simulink model "OCKModel"  (R2017b)
settings: Solver=FixedStepAuto  StartTime=0.0  StopTime=sim.T  FixedStep=sim.Ts  RelTol=1e-3
PreLoadFcn:
  | preLoadCallback
StartFcn:
  | startCallback
StopFcn:
  | stopCallback
values from neighbouring files (symbols this model uses):
  p = simulationParametersClass    [preLoadCallback.m]
undefined symbols (not defined in the file or in its folder): env, faults, plant
libraries: lowLevel x24, controllers x1, simulink x1, controllerComponents x1, flowVariants x1
settings Model: SimulationMode=rapid-accelerator  PauseTimes=78.131  SnapshotBufferSize=2  SnapshotInterval=1  ExtModeTrigDuration=100  Creator=M.Cobb  LastModifiedBy=mitch
settings DataIOCC: SaveOutput=off  StateSaveName=tmp_raccel_xout
settings OptimizationCC: DefaultParameterBehavior=Inlined  EfficientMapNaN2IntZero=off
settings DebuggingCC: InheritedTsInSrcMsg=none  AllowedUnitSystems=SI,SI (extended)
settings HardwareCC: TargetBitPerPointer=64  TargetBitPerSizeT=64  TargetBitPerPtrDiffT=64  TargetLongLongMode=on  TargetIntDivRoundTo=Zero  TargetEndianess=LittleEndian  TargetWordSize=64  TargetHWDeviceType=MATLAB Host  ProdEqTarget=off
settings RTWCC: SystemTargetFile=raccel.tlc  TemplateMakefile=raccel_default_tmf  RTWVerbose=off  RTWUseSimCustomCode=on
settings CodeAppCC: GenerateComments=off  MaxIdLength=128  MangleLength=10  SimulinkBlockComments=off
settings RaccelTargetCC: GeneratePreprocessorConditionals=Use local settings  MultiInstanceERTCode=off  ENABLE_SLEXEC_SSBRIDGE=11  RTWCAPIParams=on

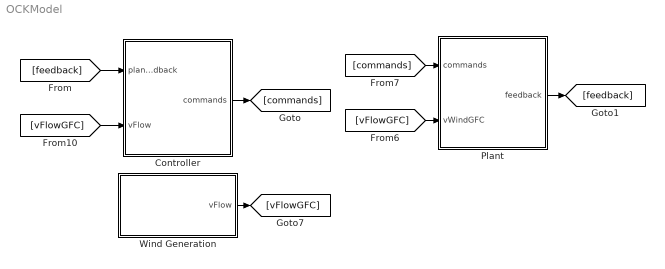
== system OCKModel ==
  Controller : Subsystem  Variant=on
  Plant : Subsystem
  Wind Generation : Subsystem
  wires:
  Wind Generation/1(vFlow) -> [vFlowGFC]
  [vFlowGFC] -> Plant/2(vWindGFC)
  [vFlowGFC] -> Controller/2(vFlow)
  Controller/1(commands) -> [commands]
  [commands] -> Plant/1(commands)
  Plant/1(feedback) -> [feedback]
  [feedback] -> Controller/1(plantFeedback)

== system OCKModel/Controller ==
  plantFeedback : Inport  OutDataTypeStr=Bus: busPlantFeedback
  vFlow : Inport  Port=2
  OCK Controller : controllers/OCK Controller  VariantControl=variantOCK
  commands : Outport  OutDataTypeStr=Bus: busControllerOutput

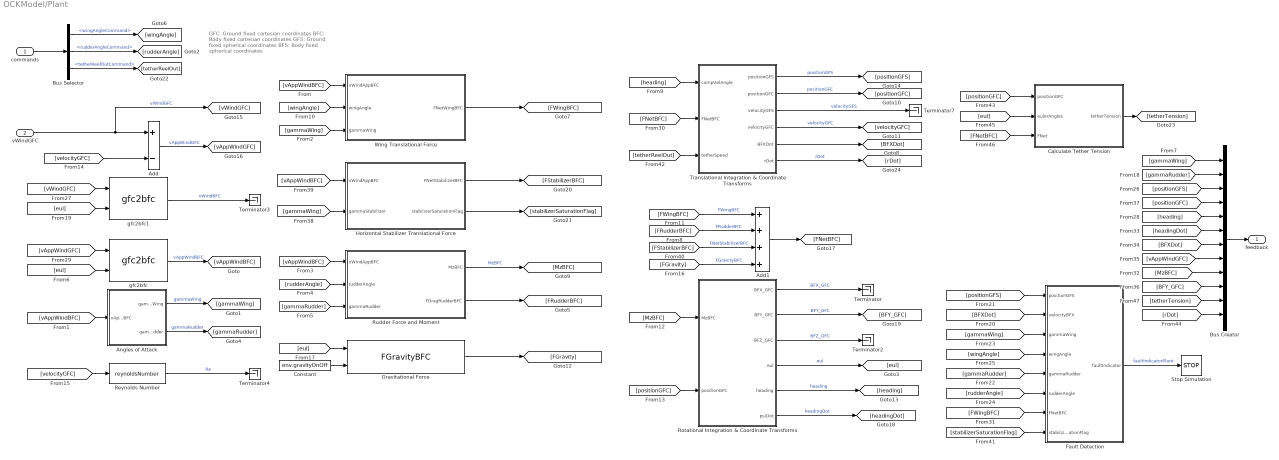
== system OCKModel/Plant ==
  note: GFC: Ground fixed cartesian coordinates
      | BFC:  Body fixed cartesian coordinates
      | GFS: Ground fixed spherical coordinates
      | BFS: Body fixed spherical coordinates
  commands : Inport  OutDataTypeStr=Bus: busControllerOutput
  vWindGFC : Inport  Port=2
  Add : Sum  Inputs=+-
  Add1 : Sum  Inputs=++++
  Angles of Attack : Subsystem
  Bus Selector : BusSelector  OutputSignals=wingAngleCommand,rudderAngleCommand,tetherReelOutCommand
  Bus Creator : BusCreator  Inputs=12  OutDataTypeStr=Bus: busPlantFeedback
  Calculate Tether Tension : Subsystem
  Constant : Constant  Value=env.gravityOnOff
  Fault Detection : Subsystem
  Gravitational Force : lowLevel/FGravityBFC
  Horizontal Stabilizer Translational Force : Subsystem
  Reynolds Number : lowLevel/reynoldsNumber
  Rotational Integration & Coordinate Transforms : Subsystem
  Rudder Force and Moment : Subsystem
  Stop Simulation : Stop
  Terminator{,2..4,7} (5 alike) : Terminator
  Translational Integration & Coordinate Transforms : Subsystem
  Wing Translational Force : Subsystem
  gfc2bfc : lowLevel/gfc2bfc
  gfc2bfc1 : lowLevel/gfc2bfc
  feedback : Outport  OutDataTypeStr=Bus: busPlantFeedback
  wires:
  vWindGFC/1 -> [vWindGFC], Add/1  "vWindGFC"
  [vAppWindBFC] -> Angles of Attack/1(vAppWindBFC)
  Angles of Attack/1(gammaWing) -> [gammaWing]  "gammaWing"
  [vAppWindBFC] -> Wing Translational Force/1(vWindAppBFC)
  Add/1 -> [vAppWindGFC]  "vAppWindGFC"
  [vAppWindBFC] -> Rudder Force and Moment/1(vWindAppBFC)
  [rudderAngle] -> Rudder Force and Moment/2(rudderAngle)
  Translational Integration & Coordinate Transforms/2(positionGFC) -> [positionGFC]  "positionGFC"
  Rudder Force and Moment/2(FDragRudderBFC) -> [FRudderBFC]
  [gammaWing] -> Wing Translational Force/3(gammaWing)
  [heading] -> Translational Integration & Coordinate Transforms/1(compVelAngle)
  Angles of Attack/2(gammaRudder) -> [gammaRudder]  "gammaRudder"
  [gammaRudder] -> Rudder Force and Moment/3(gammaRudder)
  Wing Translational Force/1(FNetWingBFC) -> [FWingBFC]
  [wingAngle] -> Wing Translational Force/2(wingAngle)
  [FNetBFC] -> Translational Integration & Coordinate Transforms/2(FNetBFC)
  Rudder Force and Moment/1(MzBFC) -> [MzBFC]  "MzBFC"
  [MzBFC] -> Rotational Integration & Coordinate Transforms/1(MzBFC)
  [positionGFC] -> Rotational Integration & Coordinate Transforms/2(positionGFC)
  Rotational Integration & Coordinate Transforms/4(eul) -> [eul]  "eul"
  Rotational Integration & Coordinate Transforms/1(BFX_GFC) -> Terminator/1  "BFX_GFC"
  Rotational Integration & Coordinate Transforms/2(BFY_GFC) -> [BFY_GFC]  "BFY_GFC"
  Rotational Integration & Coordinate Transforms/3(BFZ_GFC) -> Terminator2/1  "BFZ_GFC"
  Translational Integration & Coordinate Transforms/4(velocityGFC) -> [velocityGFC]  "velocityGFC"
  [velocityGFC] -> Add/2
  [velocityGFC] -> Reynolds Number/1
  Reynolds Number/1 -> Terminator4/1  "Re"
  Gravitational Force/1 -> [FGravity]
  [eul] -> Gravitational Force/1
  Translational Integration & Coordinate Transforms/1(positionGFS) -> [positionGFS]  "positionGFS"
  Translational Integration & Coordinate Transforms/3(velocityGFS) -> Terminator7/1  "velocityGFS"
  [eul] -> gfc2bfc1/2
  gfc2bfc1/1 -> Terminator3/1  "vWindBFC"
  Rotational Integration & Coordinate Transforms/5(heading) -> [heading]  "heading"
  Constant/1 -> Gravitational Force/2
  Translational Integration & Coordinate Transforms/5(BFXDot) -> [BFXDot]
  [BFXDot] -> Fault Detection/2(velocityBFX)
  [positionGFS] -> Fault Detection/1(positionGFS)
  Fault Detection/1(faultIndicator) -> Stop Simulation/1  "faultIndicatorPlant"
  [gammaRudder] -> Fault Detection/5(gammaRudder)
  [gammaWing] -> Fault Detection/3(gammaWing)
  [rudderAngle] -> Fault Detection/6(rudderAngle)
  [wingAngle] -> Fault Detection/4(wingAngle)
  [vWindGFC] -> gfc2bfc1/1
  gfc2bfc/1 -> [vAppWindBFC]  "vAppWindBFC"
  [eul] -> gfc2bfc/2
  [vAppWindGFC] -> gfc2bfc/1
  [FWingBFC] -> Add1/1  "FWingBFC"
  [FRudderBFC] -> Add1/2  "FRudderBFC"
  Add1/1 -> [FNetBFC]
  [FWingBFC] -> Fault Detection/7(FNetBFC)
  commands/1 -> Bus Selector/1
  Bus Selector/1 -> [wingAngle]  "<wingAngleCommand>"
  Bus Selector/2 -> [rudderAngle]  "<rudderAngleCommand>"
  [gammaWing] -> Bus Creator/1
  Bus Creator/1 -> feedback/1
  [gammaRudder] -> Bus Creator/2
  [positionGFS] -> Bus Creator/3
  Rotational Integration & Coordinate Transforms/6(psiDot) -> [headingDot]  "headingDot"
  [BFY_GFC] -> Bus Creator/10
  [MzBFC] -> Bus Creator/9
  [vAppWindGFC] -> Bus Creator/8
  [headingDot] -> Bus Creator/6
  [heading] -> Bus Creator/5
  [BFXDot] -> Bus Creator/7
  [positionGFC] -> Bus Creator/4
  [gammaWing] -> Horizontal Stabilizer Translational Force/2(gammaStabilizer)
  [vAppWindBFC] -> Horizontal Stabilizer Translational Force/1(vWindAppBFC)
  Horizontal Stabilizer Translational Force/1(FNetStabilizerBFC) -> [FStabilizerBFC]
  [FStabilizerBFC] -> Add1/3  "FNetStabilizerBFC"
  [FGravity] -> Add1/4  "FGravityBFC"
  Horizontal Stabilizer Translational Force/2(stabilizerSaturationFlag) -> [stabilizerSaturationFlag]
  [stabilizerSaturationFlag] -> Fault Detection/8(stabilizerSaturationFlag)
  Bus Selector/3 -> [tetherReelOut]  "<tetherReelOutCommand>"
  [tetherReelOut] -> Translational Integration & Coordinate Transforms/3(tetherSpeed)
  [positionGFC] -> Calculate Tether Tension/1(positionGFC)
  [eul] -> Calculate Tether Tension/2(eulerAngles)
  [FNetBFC] -> Calculate Tether Tension/3(FNet)
  [tetherTension] -> Bus Creator/11
  Calculate Tether Tension/1(tetherTension) -> [tetherTension]
  Translational Integration & Coordinate Transforms/6(rDot) -> [rDot]  "rDot"
  [rDot] -> Bus Creator/12

== system OCKModel/Wind Generation ==
  Variant Subsystem : Subsystem  Variant=on
  vFlow : Outport
  wires:
  Variant Subsystem/1(vFlowGFC) -> vFlow/1  "vFlowGFC"

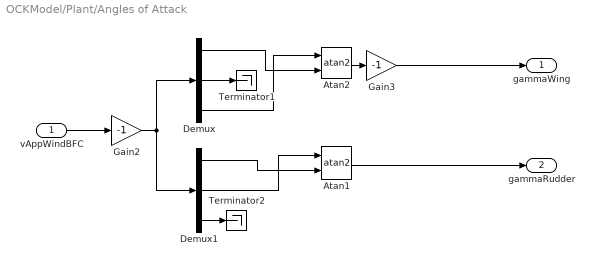
== system OCKModel/Plant/Angles of Attack ==
  vAppWindBFC : Inport
  Atan1 : Trigonometry  Operator=atan2
  Atan2 : Trigonometry  Operator=atan2
  Demux : Demux  Outputs=3
  Demux1 : Demux  Outputs=3
  Gain2 : Gain  Gain=-1
  Gain3 : Gain  Gain=-1
  Terminator1 : Terminator
  Terminator2 : Terminator
  gammaWing : Outport
  gammaRudder : Outport  Port=2
  wires:
  vAppWindBFC/1 -> Gain2/1
  Demux/1 -> Atan2/2
  Atan2/1 -> Gain3/1
  Demux/3 -> Atan2/1
  Demux/2 -> Terminator1/1
  Demux1/3 -> Terminator2/1
  Gain2/1 -> Demux1/1, Demux/1
  Atan1/1 -> gammaRudder/1
  Gain3/1 -> gammaWing/1
  Demux1/1 -> Atan1/2
  Demux1/2 -> Atan1/1

== system OCKModel/Plant/Calculate Tether Tension ==
  positionGFC : Inport
  eulerAngles : Inport  Port=2
  FNet : Inport  Port=3
  Dot Product : DotProduct  InputSameDT=on  OutDataTypeStr=Inherit: Inherit via internal rule
  gfc2bfc : lowLevel/gfc2bfc
  normalize : lowLevel/normalize
  tetherTension : Outport
  wires:
  positionGFC/1 -> normalize/1
  normalize/1 -> gfc2bfc/1
  eulerAngles/1 -> gfc2bfc/2
  FNet/1 -> Dot Product/2
  gfc2bfc/1 -> Dot Product/1
  Dot Product/1 -> tetherTension/1  "tetherTension"

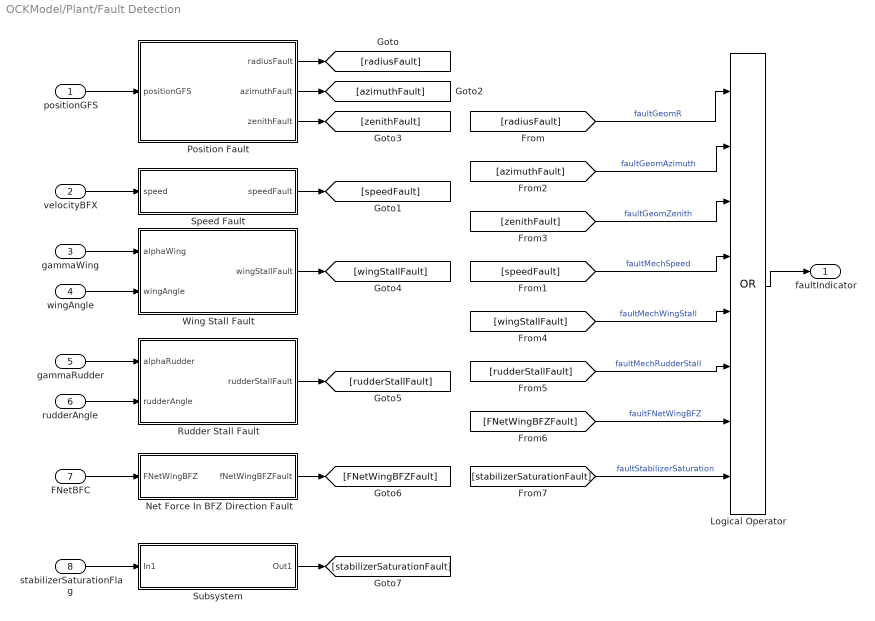
== system OCKModel/Plant/Fault Detection ==
  positionGFS : Inport
  velocityBFX : Inport  Port=2
  gammaWing : Inport  Port=3
  wingAngle : Inport  Port=4
  gammaRudder : Inport  Port=5
  rudderAngle : Inport  Port=6
  FNetBFC : Inport  Port=7
  stabilizerSaturationFlag : Inport  Port=8
  Logical Operator : Logic  Operator=OR  Inputs=8  AllPortsSameDT=off  OutDataTypeStr=boolean
  Net Force In BFZ Direction Fault : Subsystem
  Position Fault : Subsystem
  Rudder Stall Fault : Subsystem
  Speed Fault : Subsystem
  Subsystem : Subsystem
  Wing Stall Fault : Subsystem
  faultIndicator : Outport
  wires:
  positionGFS/1 -> Position Fault/1(positionGFS)
  Logical Operator/1 -> faultIndicator/1
  Speed Fault/1(speedFault) -> [speedFault]
  velocityBFX/1 -> Speed Fault/1(speed)
  [radiusFault] -> Logical Operator/1  "faultGeomR"
  [speedFault] -> Logical Operator/4  "faultMechSpeed"
  [azimuthFault] -> Logical Operator/2  "faultGeomAzimuth"
  [zenithFault] -> Logical Operator/3  "faultGeomZenith"
  Wing Stall Fault/1(wingStallFault) -> [wingStallFault]
  gammaWing/1 -> Wing Stall Fault/1(alphaWing)
  gammaRudder/1 -> Rudder Stall Fault/1(alphaRudder)
  [wingStallFault] -> Logical Operator/5  "faultMechWingStall"
  [rudderStallFault] -> Logical Operator/6  "faultMechRudderStall"
  wingAngle/1 -> Wing Stall Fault/2(wingAngle)
  rudderAngle/1 -> Rudder Stall Fault/2(rudderAngle)
  Rudder Stall Fault/1(rudderStallFault) -> [rudderStallFault]
  Position Fault/1(radiusFault) -> [radiusFault]
  Position Fault/2(azimuthFault) -> [azimuthFault]
  Position Fault/3(zenithFault) -> [zenithFault]
  Net Force In BFZ Direction Fault/1(fNetWingBFZFault) -> [FNetWingBFZFault]
  FNetBFC/1 -> Net Force In BFZ Direction Fault/1(FNetWingBFZ)
  [FNetWingBFZFault] -> Logical Operator/7  "faultFNetWingBFZ"
  [stabilizerSaturationFault] -> Logical Operator/8  "faultStabilizerSaturation"
  stabilizerSaturationFlag/1 -> Subsystem/1(In1)
  Subsystem/1(Out1) -> [stabilizerSaturationFault]

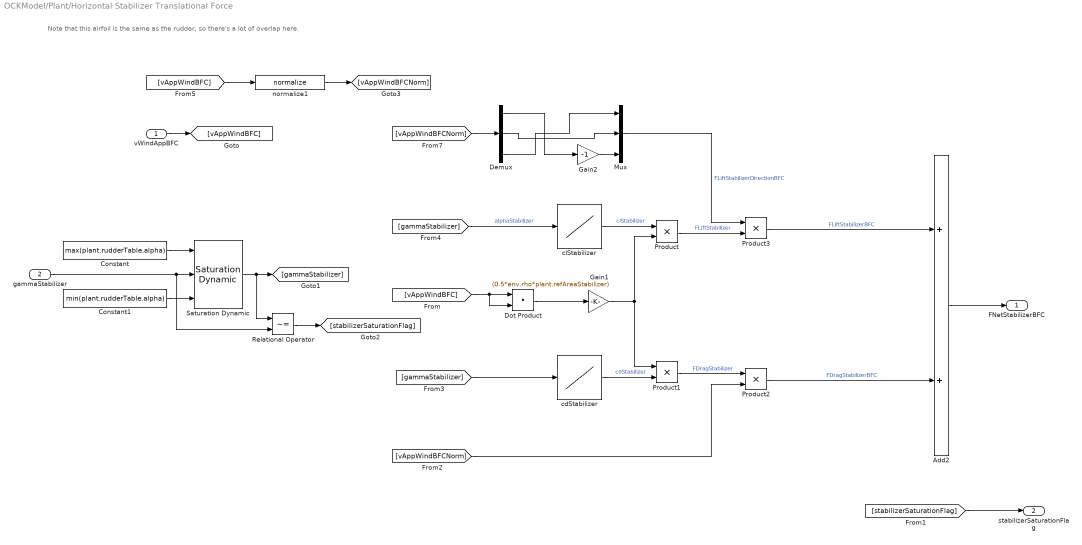
== system OCKModel/Plant/Horizontal Stabilizer Translational Force ==
  note: Note that this airfoil is the same as the rudder, so there's a lot of overlap here.
  vWindAppBFC : Inport
  gammaStabilizer : Inport  Port=2
  Add2 : Sum
  Constant : Constant  Value=max(plant.rudderTable.alpha)
  Constant1 : Constant  Value=min(plant.rudderTable.alpha)
  Demux : Demux  Outputs=3
  Dot Product : DotProduct  InputSameDT=on  OutDataTypeStr=Inherit: Inherit via internal rule
  Gain1 : Gain  Gain=(0.5*env.rho*plant.refAreaStabilizer)
  Gain2 : Gain  Gain=-1
  Mux : Mux  Inputs=3
  Product{,1..3} (4 alike) : Product
  Relational Operator : RelationalOperator  Operator=~=  OutDataTypeStr=boolean  RndMeth=Simplest
  Saturation Dynamic : simulink/Discontinuities/Saturation Dynamic  OutMin=[]  OutMax=[]  OutDataTypeStr=Inherit: Same as second input  OutDataType=fixdt(1, 16)  OutScaling=2^-10  DoSatur=off
  cdStabilizer : Lookup_n-D  NumberOfTableDimensions=1  BreakpointsForDimension1=plant.rudderTable.alpha  Table=plant.rudderTable.cd  InternalRulePriority=Speed  RndMeth=Simplest  InputSameDT=on
  clStabilizer : Lookup_n-D  NumberOfTableDimensions=1  BreakpointsForDimension1=plant.rudderTable.alpha  Table=plant.rudderTable.cl  InternalRulePriority=Speed  RndMeth=Simplest  InputSameDT=on
  normalize1 : lowLevel/normalize
  FNetStabilizerBFC : Outport
  stabilizerSaturationFlag : Outport  Port=2
  wires:
  Product1/1 -> Product2/1  "FDragStabilizer"
  Product2/1 -> Add2/2  "FDragStabilizerBFC"
  Product/1 -> Product3/2  "FLiftStabilizer"
  Product3/1 -> Add2/1  "FLiftStabilizerBFC"
  Dot Product/1 -> Gain1/1
  clStabilizer/1 -> Product/1  "clStabilizer"
  [vAppWindBFC] -> Dot Product/1, Dot Product/2
  Gain1/1 -> Product/2, Product1/1
  cdStabilizer/1 -> Product1/2  "cdStabilizer"
  vWindAppBFC/1 -> [vAppWindBFC]
  gammaStabilizer/1 -> Relational Operator/2, Saturation Dynamic/2
  Demux/2 -> Mux/2
  Demux/1 -> Gain2/1
  Mux/1 -> Product3/1  "FLiftStabilizerDirectionBFC"
  Demux/3 -> Mux/1
  [vAppWindBFC] -> normalize1/1
  normalize1/1 -> [vAppWindBFCNorm]
  [vAppWindBFCNorm] -> Demux/1
  [vAppWindBFCNorm] -> Product2/2
  Gain2/1 -> Mux/3
  [gammaStabilizer] -> cdStabilizer/1
  [gammaStabilizer] -> clStabilizer/1  "alphaStabilizer"
  Saturation Dynamic/1 -> Relational Operator/1, [gammaStabilizer]
  Constant/1 -> Saturation Dynamic/1
  Constant1/1 -> Saturation Dynamic/3
  Relational Operator/1 -> [stabilizerSaturationFlag]
  [stabilizerSaturationFlag] -> stabilizerSaturationFlag/1
  Add2/1 -> FNetStabilizerBFC/1

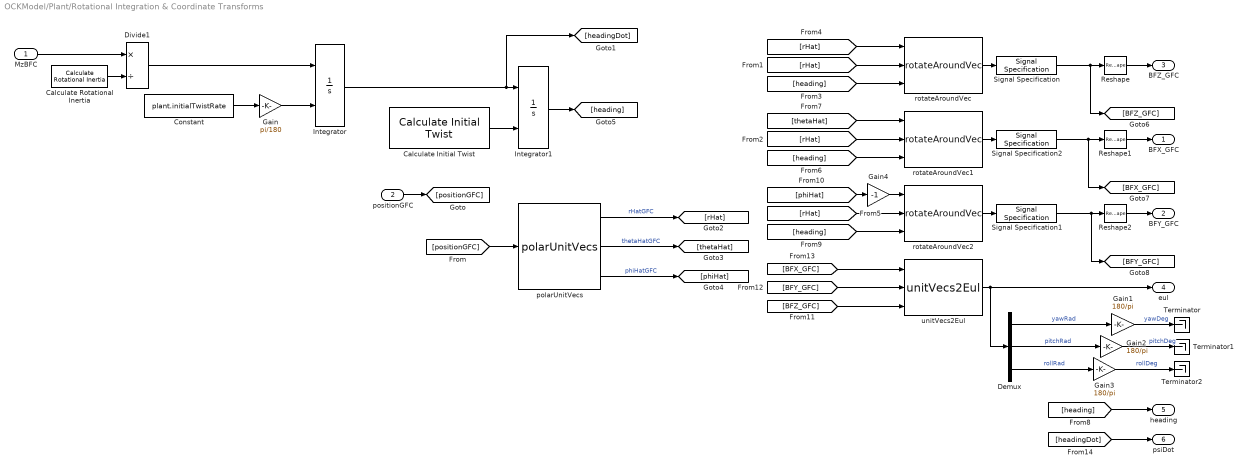
== system OCKModel/Plant/Rotational Integration & Coordinate Transforms ==
  MzBFC : Inport  PortDimensions=1
  positionGFC : Inport  Port=2
  Calculate Rotational Inertia : lowLevel/Calculate Rotational Inertia
  Calculate Initial Twist : controllerComponents/Calculate Initial Twist
  Constant : Constant  Value=plant.initialTwistRate
  Demux : Demux  Outputs=3
  Divide1 : Product  Inputs=*/
  Gain : Gain  Gain=pi/180
  Gain1 : Gain  Gain=180/pi
  Gain2 : Gain  Gain=180/pi
  Gain3 : Gain  Gain=180/pi
  Gain4 : Gain  Gain=-1
  Integrator : Integrator  InitialConditionSource=external  InitialCondition=plant.initialTwistRate
  Integrator1 : Integrator  InitialConditionSource=external  InitialCondition=plant.initialTwist
  Reshape : Reshape  OutputDimensions=[3 1]
  Reshape1 : Reshape  OutputDimensions=[3 1]
  Reshape2 : Reshape  OutputDimensions=[3 1]
  Signal Specification : SignalSpecification  Dimensions=[1 3]
  Signal Specification1 : SignalSpecification  Dimensions=[1 3]
  Signal Specification2 : SignalSpecification  Dimensions=[1 3]
  Terminator : Terminator
  Terminator1 : Terminator
  Terminator2 : Terminator
  polarUnitVecs : lowLevel/polarUnitVecs
  rotateAroundVec : lowLevel/rotateAroundVec
  rotateAroundVec1 : lowLevel/rotateAroundVec
  rotateAroundVec2 : lowLevel/rotateAroundVec
  unitVecs2Eul : lowLevel/unitVecs2Eul
  BFX_GFC : Outport
  BFY_GFC : Outport  Port=2
  BFZ_GFC : Outport  Port=3
  eul : Outport  Port=4  PortDimensions=3
  heading : Outport  Port=5  PortDimensions=1
  psiDot : Outport  Port=6  PortDimensions=1
  wires:
  MzBFC/1 -> Divide1/1
  Integrator/1 -> [headingDot], Integrator1/1
  positionGFC/1 -> [positionGFC]
  [positionGFC] -> polarUnitVecs/1
  polarUnitVecs/1 -> [rHat]  "rHatGFC"
  polarUnitVecs/2 -> [thetaHat]  "thetaHatGFC"
  polarUnitVecs/3 -> [phiHat]  "phiHatGFC"
  Integrator1/1 -> [heading]
  [heading] -> rotateAroundVec/3
  [rHat] -> rotateAroundVec/1
  [rHat] -> rotateAroundVec/2
  [thetaHat] -> rotateAroundVec1/1
  [heading] -> rotateAroundVec1/3
  [rHat] -> rotateAroundVec1/2
  [phiHat] -> Gain4/1
  [heading] -> rotateAroundVec2/3
  [rHat] -> rotateAroundVec2/2
  unitVecs2Eul/1 -> Demux/1, eul/1
  [BFZ_GFC] -> unitVecs2Eul/3
  [BFY_GFC] -> unitVecs2Eul/2
  [BFX_GFC] -> unitVecs2Eul/1
  Demux/3 -> Gain3/1  "rollRad"
  Demux/2 -> Gain2/1  "pitchRad"
  Demux/1 -> Gain1/1  "yawRad"
  Gain1/1 -> Terminator/1  "yawDeg"
  Gain2/1 -> Terminator1/1  "pitchDeg"
  Gain3/1 -> Terminator2/1  "rollDeg"
  Gain4/1 -> rotateAroundVec2/1
  rotateAroundVec/1 -> Signal Specification/1
  rotateAroundVec1/1 -> Signal Specification2/1
  rotateAroundVec2/1 -> Signal Specification1/1
  Signal Specification/1 -> Reshape/1, [BFZ_GFC]
  Signal Specification2/1 -> [BFX_GFC], Reshape1/1
  Signal Specification1/1 -> [BFY_GFC], Reshape2/1
  Reshape/1 -> BFZ_GFC/1
  Reshape1/1 -> BFX_GFC/1
  Reshape2/1 -> BFY_GFC/1
  [heading] -> heading/1
  [headingDot] -> psiDot/1
  Calculate Initial Twist/1 -> Integrator1/2
  Calculate Rotational Inertia/1 -> Divide1/2
  Divide1/1 -> Integrator/1
  Constant/1 -> Gain/1
  Gain/1 -> Integrator/2

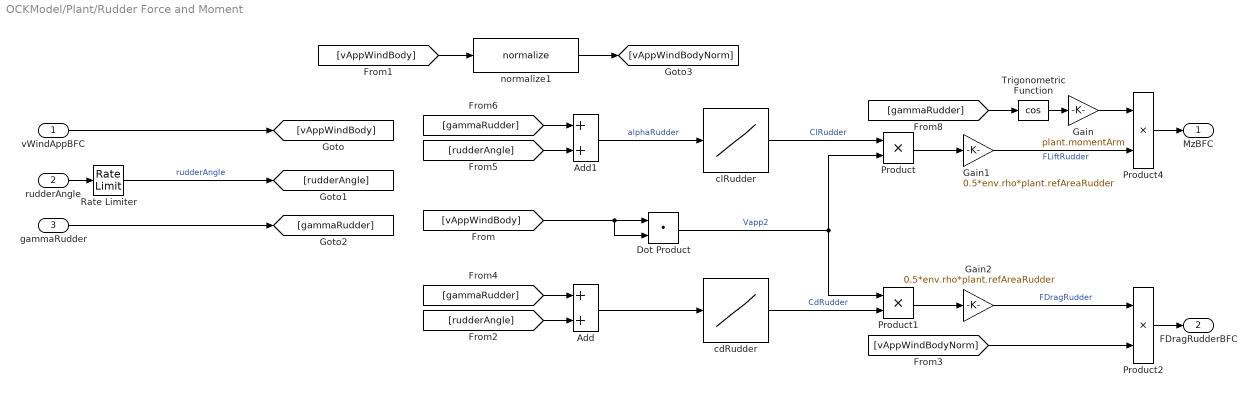
== system OCKModel/Plant/Rudder Force and Moment ==
  vWindAppBFC : Inport
  rudderAngle : Inport  Port=2
  gammaRudder : Inport  Port=3
  Add : Sum
  Add1 : Sum
  Dot Product : DotProduct  InputSameDT=on  OutDataTypeStr=Inherit: Inherit via internal rule
  Gain : Gain  Gain=plant.momentArm
  Gain1 : Gain  Gain=0.5*env.rho*plant.refAreaRudder
  Gain2 : Gain  Gain=0.5*env.rho*plant.refAreaRudder
  Product{,1..2,4} (4 alike) : Product
  Rate Limiter : RateLimiter  RisingSlewLimit=plant.rudderAngleRateLimit*pi/180  FallingSlewLimit=-plant.rudderAngleRateLimit*pi/180  SampleTimeMode=inherited
  Trigonometric Function : Trigonometry  Operator=cos
  cdRudder : Lookup_n-D  NumberOfTableDimensions=1  BreakpointsForDimension1=plant.rudderTable.alpha  Table=plant.rudderTable.cd  InternalRulePriority=Speed  RndMeth=Simplest  InputSameDT=on
  clRudder : Lookup_n-D  NumberOfTableDimensions=1  BreakpointsForDimension1=plant.rudderTable.alpha  Table=plant.rudderTable.cl  InternalRulePriority=Speed  RndMeth=Simplest  InputSameDT=on
  normalize1 : lowLevel/normalize
  MzBFC : Outport
  FDragRudderBFC : Outport  Port=2
  wires:
  clRudder/1 -> Product/1  "ClRudder"
  [vAppWindBody] -> Dot Product/2, Dot Product/1
  Dot Product/1 -> Product1/1, Product/2  "Vapp2"
  vWindAppBFC/1 -> [vAppWindBody]
  rudderAngle/1 -> Rate Limiter/1
  Product/1 -> Gain1/1
  cdRudder/1 -> Product1/2  "CdRudder"
  Product1/1 -> Gain2/1
  Gain2/1 -> Product2/1  "FDragRudder"
  [vAppWindBodyNorm] -> Product2/2
  gammaRudder/1 -> [gammaRudder]
  [rudderAngle] -> Add/2
  [gammaRudder] -> Add/1
  Add/1 -> cdRudder/1
  [rudderAngle] -> Add1/2
  [gammaRudder] -> Add1/1
  Add1/1 -> clRudder/1  "alphaRudder"
  Gain1/1 -> Product4/2  "FLiftRudder"
  [vAppWindBody] -> normalize1/1
  normalize1/1 -> [vAppWindBodyNorm]
  Product2/1 -> FDragRudderBFC/1
  [gammaRudder] -> Trigonometric Function/1
  Product4/1 -> MzBFC/1
  Trigonometric Function/1 -> Gain/1
  Gain/1 -> Product4/1
  Rate Limiter/1 -> [rudderAngle]  "rudderAngle"

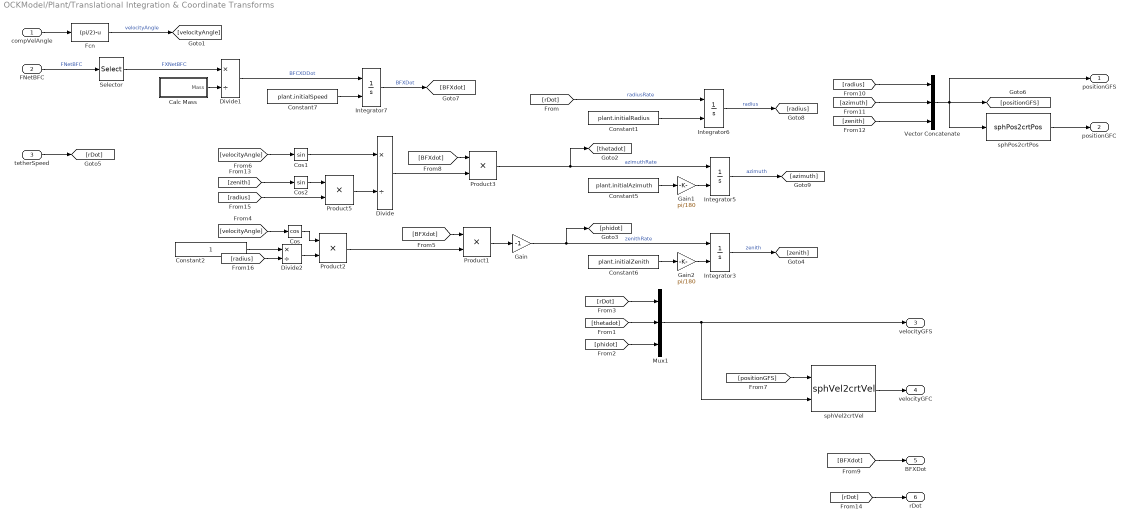
== system OCKModel/Plant/Translational Integration & Coordinate Transforms ==
  compVelAngle : Inport
  FNetBFC : Inport  Port=2
  tetherSpeed : Inport  Port=3
  Calc Mass : Subsystem
  Constant1 : Constant  Value=plant.initialRadius
  Constant2 : Constant
  Constant5 : Constant  Value=plant.initialAzimuth
  Constant6 : Constant  Value=plant.initialZenith
  Constant7 : Constant  Value=plant.initialSpeed
  Cos : Trigonometry  Operator=cos
  Cos1 : Trigonometry
  Cos2 : Trigonometry
  Divide : Product  Inputs=*/
  Divide1 : Product  Inputs=*/
  Divide2 : Product  Inputs=*/
  Fcn : Fcn  Expr=(pi/2)-u
  Gain : Gain  Gain=-1
  Gain1 : Gain  Gain=pi/180
  Gain2 : Gain  Gain=pi/180
  Integrator3 : Integrator  InitialConditionSource=external  InitialCondition=p.initPositionGFS(3)
  Integrator5 : Integrator  InitialConditionSource=external  InitialCondition=p.initPositionGFS(2)
  Integrator6 : Integrator  InitialConditionSource=external  InitialCondition=p.initPositionGFS(1)
  Integrator7 : Integrator  InitialConditionSource=external  InitialCondition=p.initVelocity
  Mux1 : Mux  Inputs=3
  Product{1..3,5} (4 alike) : Product
  Selector : Selector  InputPortWidth=3  IndexOptions=Index vector (dialog)  Indices=1  OutputSizes=1
  Vector Concatenate : Concatenate  NumInputs=3
  sphPos2crtPos : lowLevel/sphPos2crtPos
  sphVel2crtVel : lowLevel/sphVel2crtVel
  positionGFS : Outport  PortDimensions=3
  positionGFC : Outport  Port=2  PortDimensions=3
  velocityGFS : Outport  Port=3  PortDimensions=3
  velocityGFC : Outport  Port=4  PortDimensions=3
  BFXDot : Outport  Port=5
  rDot : Outport  Port=6
  wires:
  Gain/1 -> [phidot], Integrator3/1  "zenithRate"
  Integrator5/1 -> [azimuth]  "azimuth"
  Product3/1 -> [thetadot], Integrator5/1  "azimuthRate"
  Integrator3/1 -> [zenith]  "zenith"
  sphPos2crtPos/1 -> positionGFC/1
  sphVel2crtVel/1 -> velocityGFC/1
  [rDot] -> Mux1/1
  [thetadot] -> Mux1/2
  [phidot] -> Mux1/3
  FNetBFC/1 -> Selector/1  "FNetBFC"
  compVelAngle/1 -> Fcn/1
  Integrator6/1 -> [radius]  "radius"
  Mux1/1 -> sphVel2crtVel/2, velocityGFS/1
  [rDot] -> Integrator6/1  "radiusRate"
  [positionGFS] -> sphVel2crtVel/1
  Fcn/1 -> [velocityAngle]  "velocityAngle"
  [BFXdot] -> Product3/1
  [velocityAngle] -> Cos1/1
  Divide/1 -> Product3/2
  Cos1/1 -> Divide/1
  [radius] -> Product5/2
  [zenith] -> Cos2/1
  Cos2/1 -> Product5/1
  Product5/1 -> Divide/2
  [BFXdot] -> Product1/1
  [velocityAngle] -> Cos/1
  Product2/1 -> Product1/2
  Cos/1 -> Product2/1
  Divide2/1 -> Product2/2
  Product1/1 -> Gain/1
  Integrator7/1 -> [BFXdot]  "BFXDot"
  Divide1/1 -> Integrator7/1  "BFCXDDot"
  [BFXdot] -> BFXDot/1
  Constant1/1 -> Integrator6/2
  Constant5/1 -> Gain1/1
  Vector Concatenate/1 -> [positionGFS], positionGFS/1, sphPos2crtPos/1
  [radius] -> Vector Concatenate/1
  [azimuth] -> Vector Concatenate/2
  [zenith] -> Vector Concatenate/3
  Constant6/1 -> Gain2/1
  Gain1/1 -> Integrator5/2
  Gain2/1 -> Integrator3/2
  Constant7/1 -> Integrator7/2
  tetherSpeed/1 -> [rDot]
  Selector/1 -> Divide1/1  "FXNetBFC"
  Calc Mass/1(Mass) -> Divide1/2
  [rDot] -> rDot/1
  [radius] -> Divide2/2
  Constant2/1 -> Divide2/1

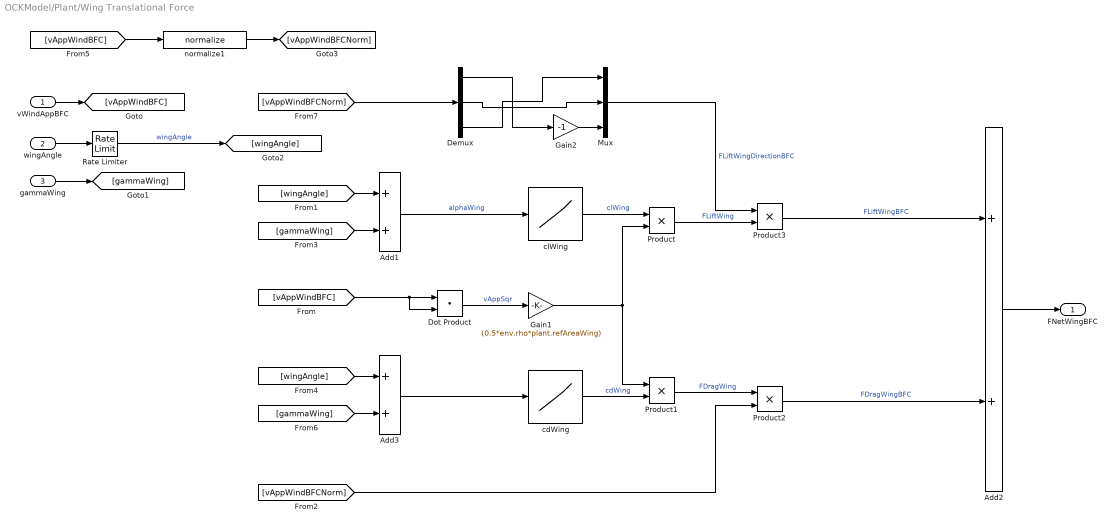
== system OCKModel/Plant/Wing Translational Force ==
  vWindAppBFC : Inport
  wingAngle : Inport  Port=2
  gammaWing : Inport  Port=3
  Add1 : Sum
  Add2 : Sum
  Add3 : Sum
  Demux : Demux  Outputs=3
  Dot Product : DotProduct  InputSameDT=on  OutDataTypeStr=Inherit: Inherit via internal rule
  Gain1 : Gain  Gain=(0.5*env.rho*plant.refAreaWing)
  Gain2 : Gain  Gain=-1
  Mux : Mux  Inputs=3
  Product{,1..3} (4 alike) : Product
  Rate Limiter : RateLimiter  RisingSlewLimit=plant.wingAngleRateLimit*pi/180  FallingSlewLimit=-plant.wingAngleRateLimit*pi/180  SampleTimeMode=inherited
  cdWing : Lookup_n-D  NumberOfTableDimensions=1  BreakpointsForDimension1=plant.wingTable.alpha  Table=plant.wingTable.cd  InternalRulePriority=Speed  RndMeth=Simplest  InputSameDT=on
  clWing : Lookup_n-D  NumberOfTableDimensions=1  BreakpointsForDimension1=plant.wingTable.alpha  Table=plant.wingTable.cl  InternalRulePriority=Speed  RndMeth=Simplest  InputSameDT=on
  normalize1 : lowLevel/normalize
  FNetWingBFC : Outport
  wires:
  Product1/1 -> Product2/1  "FDragWing"
  Product2/1 -> Add2/2  "FDragWingBFC"
  Product/1 -> Product3/2  "FLiftWing"
  Product3/1 -> Add2/1  "FLiftWingBFC"
  Dot Product/1 -> Gain1/1  "vAppSqr"
  clWing/1 -> Product/1  "clWing"
  [vAppWindBFC] -> Dot Product/2, Dot Product/1
  Gain1/1 -> Product/2, Product1/1
  cdWing/1 -> Product1/2  "cdWing"
  vWindAppBFC/1 -> [vAppWindBFC]
  Add2/1 -> FNetWingBFC/1
  gammaWing/1 -> [gammaWing]
  wingAngle/1 -> Rate Limiter/1
  [wingAngle] -> Add3/1
  [gammaWing] -> Add3/2
  Demux/1 -> Gain2/1
  Mux/1 -> Product3/1  "FLiftWingDirectionBFC"
  Demux/3 -> Mux/1
  [vAppWindBFC] -> normalize1/1
  normalize1/1 -> [vAppWindBFCNorm]
  [vAppWindBFCNorm] -> Demux/1
  [vAppWindBFCNorm] -> Product2/2
  Gain2/1 -> Mux/3
  Add3/1 -> cdWing/1
  [wingAngle] -> Add1/1
  [gammaWing] -> Add1/2
  Add1/1 -> clWing/1  "alphaWing"
  Rate Limiter/1 -> [wingAngle]  "wingAngle"
  Demux/2 -> Mux/2

== system OCKModel/Wind Generation/Variant Subsystem ==
  Constant Wind : flowVariants/Constant Wind  VariantControl=variantConstant
  vFlowGFC : Outport

== system OCKModel/Plant/Fault Detection/Net Force In BFZ Direction Fault ==
  note: If net force in body fixed Z direction is zero or negative
  FNetWingBFZ : Inport
  Constant10 : Constant  Value=faults.forceZHigh
  Constant11 : Constant  Value=faults.forceZEnable
  Constant9 : Constant  Value=faults.forceZLow
  Out Of Bounds Fault : lowLevel/Out Of Bounds Fault
  Selector : Selector  InputPortWidth=3  IndexOptions=Index vector (dialog)  Indices=3  OutputSizes=1
  fNetWingBFZFault : Outport
  wires:
  FNetWingBFZ/1 -> Selector/1
  Selector/1 -> Out Of Bounds Fault/1
  Constant9/1 -> Out Of Bounds Fault/2
  Constant10/1 -> Out Of Bounds Fault/3
  Constant11/1 -> Out Of Bounds Fault/4
  Out Of Bounds Fault/1 -> fNetWingBFZFault/1

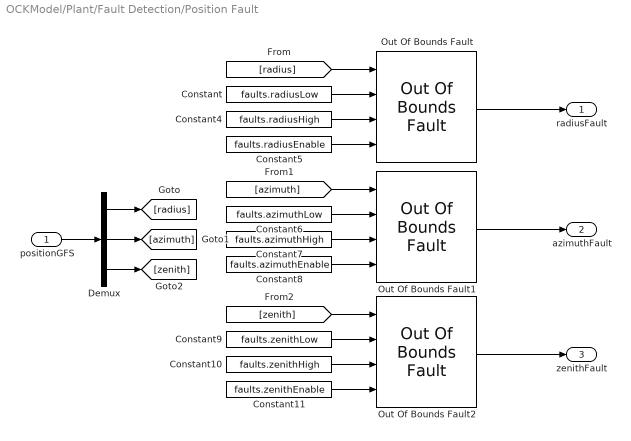
== system OCKModel/Plant/Fault Detection/Position Fault ==
  positionGFS : Inport
  Constant : Constant  Value=faults.radiusLow
  Constant10 : Constant  Value=faults.zenithHigh
  Constant11 : Constant  Value=faults.zenithEnable
  Constant4 : Constant  Value=faults.radiusHigh
  Constant5 : Constant  Value=faults.radiusEnable
  Constant6 : Constant  Value=faults.azimuthLow
  Constant7 : Constant  Value=faults.azimuthHigh
  Constant8 : Constant  Value=faults.azimuthEnable
  Constant9 : Constant  Value=faults.zenithLow
  Demux : Demux  Outputs=3
  Out Of Bounds Fault : lowLevel/Out Of Bounds Fault
  Out Of Bounds Fault1 : lowLevel/Out Of Bounds Fault
  Out Of Bounds Fault2 : lowLevel/Out Of Bounds Fault
  radiusFault : Outport
  azimuthFault : Outport  Port=2
  zenithFault : Outport  Port=3
  wires:
  positionGFS/1 -> Demux/1
  Out Of Bounds Fault/1 -> radiusFault/1
  Out Of Bounds Fault1/1 -> azimuthFault/1
  Out Of Bounds Fault2/1 -> zenithFault/1
  Demux/1 -> [radius]
  Demux/2 -> [azimuth]
  Demux/3 -> [zenith]
  [radius] -> Out Of Bounds Fault/1
  [azimuth] -> Out Of Bounds Fault1/1
  [zenith] -> Out Of Bounds Fault2/1
  Constant/1 -> Out Of Bounds Fault/2
  Constant5/1 -> Out Of Bounds Fault/4
  Constant4/1 -> Out Of Bounds Fault/3
  Constant7/1 -> Out Of Bounds Fault1/3
  Constant6/1 -> Out Of Bounds Fault1/2
  Constant8/1 -> Out Of Bounds Fault1/4
  Constant9/1 -> Out Of Bounds Fault2/2
  Constant10/1 -> Out Of Bounds Fault2/3
  Constant11/1 -> Out Of Bounds Fault2/4

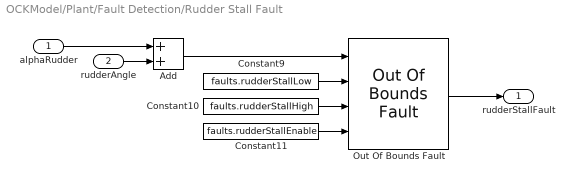
== system OCKModel/Plant/Fault Detection/Rudder Stall Fault ==
  alphaRudder : Inport
  rudderAngle : Inport  Port=2
  Add : Sum
  Constant10 : Constant  Value=faults.rudderStallHigh
  Constant11 : Constant  Value=faults.rudderStallEnable
  Constant9 : Constant  Value=faults.rudderStallLow
  Out Of Bounds Fault : lowLevel/Out Of Bounds Fault
  rudderStallFault : Outport
  wires:
  rudderAngle/1 -> Add/2
  alphaRudder/1 -> Add/1
  Out Of Bounds Fault/1 -> rudderStallFault/1
  Constant9/1 -> Out Of Bounds Fault/2
  Constant11/1 -> Out Of Bounds Fault/4
  Constant10/1 -> Out Of Bounds Fault/3
  Add/1 -> Out Of Bounds Fault/1

== system OCKModel/Plant/Fault Detection/Speed Fault ==
  note: If body fixed speed in x is negative
  speed : Inport
  Constant10 : Constant  Value=faults.speedHigh
  Constant11 : Constant  Value=faults.speedEnable
  Constant9 : Constant  Value=faults.speedLow
  Out Of Bounds Fault : lowLevel/Out Of Bounds Fault
  speedFault : Outport
  wires:
  speed/1 -> Out Of Bounds Fault/1
  Constant9/1 -> Out Of Bounds Fault/2
  Constant10/1 -> Out Of Bounds Fault/3
  Constant11/1 -> Out Of Bounds Fault/4
  Out Of Bounds Fault/1 -> speedFault/1

== system OCKModel/Plant/Fault Detection/Subsystem ==
  In1 : Inport
  Constant : Constant  Value=0  OutDataTypeStr=boolean
  Constant1 : Constant  Value=faults.stabilizerSaturationEnable  OutDataTypeStr=boolean
  Multiport Switch : MultiPortSwitch  DataPortOrder=Zero-based contiguous  Inputs=2
  Out1 : Outport
  wires:
  Constant/1 -> Multiport Switch/2
  Multiport Switch/1 -> Out1/1
  In1/1 -> Multiport Switch/3
  Constant1/1 -> Multiport Switch/1

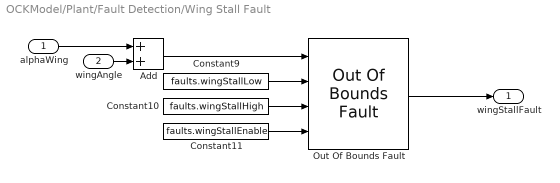
== system OCKModel/Plant/Fault Detection/Wing Stall Fault ==
  alphaWing : Inport
  wingAngle : Inport  Port=2
  Add : Sum
  Constant10 : Constant  Value=faults.wingStallHigh
  Constant11 : Constant  Value=faults.wingStallEnable
  Constant9 : Constant  Value=faults.wingStallLow
  Out Of Bounds Fault : lowLevel/Out Of Bounds Fault
  wingStallFault : Outport
  wires:
  alphaWing/1 -> Add/1
  wingAngle/1 -> Add/2
  Out Of Bounds Fault/1 -> wingStallFault/1
  Constant11/1 -> Out Of Bounds Fault/4
  Constant10/1 -> Out Of Bounds Fault/3
  Constant9/1 -> Out Of Bounds Fault/2
  Add/1 -> Out Of Bounds Fault/1

== system OCKModel/Plant/Translational Integration & Coordinate Transforms/Calc Mass ==
  Add1 : Sum
  Constant1 : Constant  Value=plant.addedMassMultiplier
  Constant2 : Constant  Value=plant.mass
  Constant4 : Constant  Value=env.rho
  Product3 : Product
  Mass : Outport
  wires:
  Constant4/1 -> Product3/1
  Add1/1 -> Mass/1
  Product3/1 -> Add1/1
  Constant2/1 -> Add1/2
  Constant1/1 -> Product3/2
